simulink model "model"  (R2025b)
settings: Solver=VariableStepAuto  StartTime=0.0  StopTime=10.0  RelTol=1e-3
values from neighbouring files (symbols this model uses):
  A_inv = 1/ A    (= 0.25)    [script.m]
  k_valve = S * sqrt(2 * g)    [script.m]
  Qin = 10 / 1000    (= 0.01)    [script.m]
settings Model: Creator=Vladimir  LastModifiedBy=Vladimir

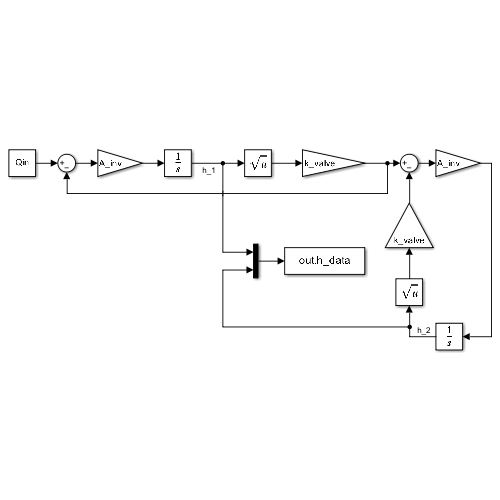
[thumbnail: Simulink's stored preview of the top-level diagram]
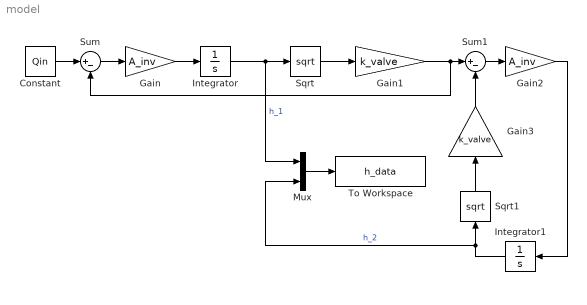
== system model ==
  Constant : Constant  Value=Qin
  Gain : Gain  Gain=A_inv
  Gain1 : Gain  Gain=k_valve
  Gain2 : Gain  Gain=A_inv
  Gain3 : Gain  Gain=k_valve
  Integrator : Integrator
  Integrator1 : Integrator
  Mux : Mux  Inputs=2
  Sqrt : Sqrt
  Sqrt1 : Sqrt
  Sum : Sum  Inputs=|+-
  Sum1 : Sum  Inputs=|+-
  To Workspace : ToWorkspace  VariableName=h_data  SaveFormat=Timeseries  SampleTime=-1
  wires:
  Constant/1 -> Sum/1
  Sum/1 -> Gain/1
  Gain/1 -> Integrator/1
  Integrator/1 -> Sqrt/1, Mux/1  "h_1"
  Sqrt/1 -> Gain1/1
  Gain1/1 -> Sum/2, Sum1/1
  Sum1/1 -> Gain2/1
  Gain2/1 -> Integrator1/1
  Integrator1/1 -> Mux/2, Sqrt1/1  "h_2"
  Sqrt1/1 -> Gain3/1
  Gain3/1 -> Sum1/2
  Mux/1 -> To Workspace/1
